simulink model "double_pendulum_model"  (R2020a)
settings: Solver=VariableStepAuto  StartTime=0.0  StopTime=10.0  RelTol=1e-3
values from neighbouring files (symbols this model uses):
  l = 1    [pend4par.m]    (also in pendcartpar.m; pendragpar.m = 0.1)
  m = 1    [cannonballpar.m]    (also in pendcartpar.m; pendragpar.m = 0.01)
undefined symbols (not defined in the file or in its folder): double_pendulum
settings Model: Creator=Tomo  LastModifiedBy=Tomo

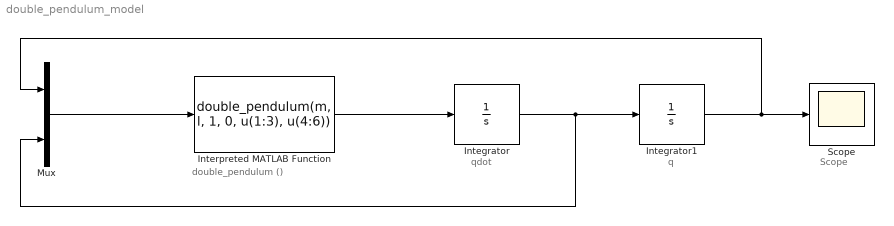
== system double_pendulum_model ==
  note: Scope
  note: double_pendulum ()
  note: qdot
  note: q
  Integrator : Integrator
  Integrator1 : Integrator
  Interpreted MATLAB Function : MATLABFcn  MATLABFcn=double_pendulum(m, l, 1, 0, u(1:3), u(4:6))  OutputDimensions=3  OutputSignalType=real
  Mux : Mux  Inputs=2
  Scope : Scope
  wires:
  Mux/1 -> Interpreted MATLAB Function/1
  Interpreted MATLAB Function/1 -> Integrator/1
  Integrator/1 -> Mux/2, Integrator1/1
  Integrator1/1 -> Mux/1, Scope/1
